simulink model "orbitcom_R20b_finalversion"  (R2020b)
settings: Solver=FixedStepAuto  StartTime=0.0  StopTime=tsimulation  FixedStep=delta_t  RelTol=1e-3
values from neighbouring files (symbols this model uses):
  a = 6678    [linkbudgetuplinkvhf.m]    (also in main_link.m)
  d_0 = (sqrt((R_earth+alt_orbit)^2-R_earth^2))/1000    [linkbudgetuplinkvhf.m]    (also in main_link.m)
  day = 1    [main_link.m]
  delta_t = 0.5    [main_link.m]
  e = 0.001    [main_link.m]
  h = u(1)/1000    [ecef_2_enu.m]    (also in geod_2_ecef.m = u(1); main_link.m = 189)
  hours = 4    [main_link.m]
  i = 51.6    [main_link.m]
  lat = u(2)    [ecef_2_enu.m]    (also in geod_2_ecef.m; main_link.m = 43.6)
  long = u(3)    [ecef_2_enu.m]    (also in geod_2_ecef.m; main_link.m = 1.44)
  m = 10    [main_link.m]
  minutes = 0    [main_link.m]
  month = 1    [main_link.m]
  nu = 0    [main_link.m]
  O = 120    [main_link.m]
  o = 90    [main_link.m]
  seconds = 0    [main_link.m]
  year = 2020    [main_link.m]
undefined symbols (not defined in the file or in its folder): DiscIntNeverNeededParam, km, s
libraries: vrlib x10, aerolibutil x9, aerolibconvert2 x6, sharedtransform x1, My_library x1, simulink_extras x1, aerolibgravity2 x1, aerolibcelestial x1
settings Model: Creator=Ricardo  LastModifiedBy=bouza

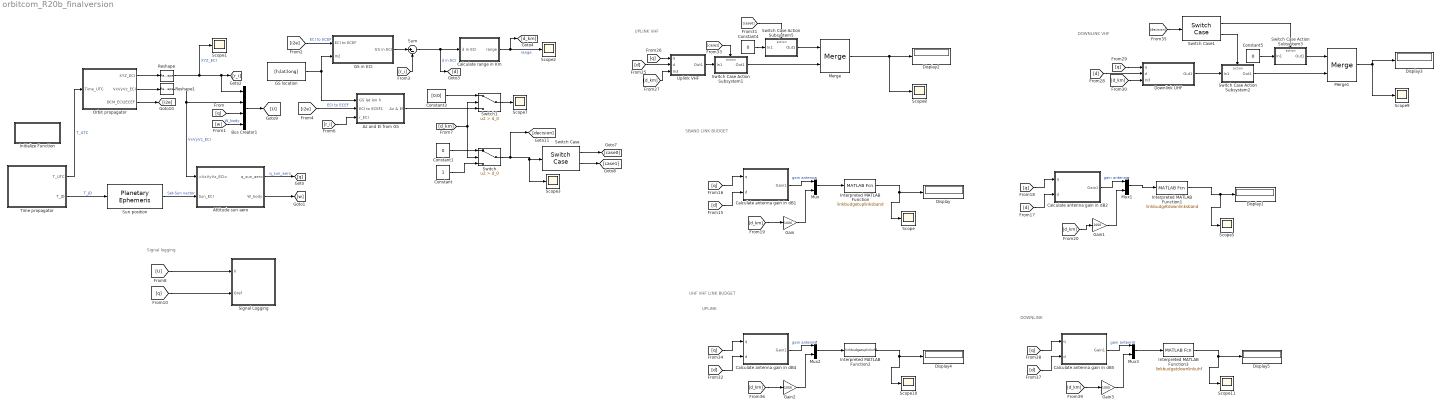
== system orbitcom_R20b_finalversion ==
  note: UHF VHF LINK BUDGET
  note: SBAND LINK BUDGET
  note: UPLINK VHF
  note: Signal logging
  note: DOWNLINK VHF
  note: UPLINK
  note: DOWNLINK
  Attitude sun aero : Subsystem
  Az and El from GS : Subsystem
  Bus Creator1 : BusCreator  Inputs=4
  Calculate antenna gain in dB1 : Subsystem
  Calculate antenna gain in dB2 : Subsystem
  Calculate antenna gain in dB4 : Subsystem
  Calculate antenna gain in dB5 : Subsystem
  Calculate range in Km : Subsystem
  Constant : Constant
  Constant1 : Constant  Value=0
  Constant3 : Constant  Value=[0;0]
  Constant4 : Constant  Value=0
  Constant5 : Constant  Value=0
  Display{,1..5} (6 alike) : Display
  Downlink UHF : Subsystem
  GS in ECI : Subsystem
  GS location : Constant  Value=[h;lat;long]
  Gain{,1..3} (4 alike) : Gain  Gain=1000
  Initialize Function : Subsystem  TreatAsAtomicUnit=on
  Interpreted MATLAB Function : MATLABFcn  MATLABFcn=linkbudgetuplinksband  OutputDimensions=1
  Interpreted MATLAB Function1 : MATLABFcn  MATLABFcn=linkbudgetdownlinksband  OutputDimensions=1
  Interpreted MATLAB Function2 : MATLABFcn  MATLABFcn=linkbudgetuplinkvhf  OutputDimensions=1
  Interpreted MATLAB Function3 : MATLABFcn  MATLABFcn=linkbudgetdownlinkuhf  OutputDimensions=1
  Merge : Merge
  Merge1 : Merge
  Mux{,1..3} (4 alike) : Mux  Inputs=2
  Orbit propagator : Subsystem
  Reshape : Reshape
  Reshape1 : Reshape
  Scope{,1..3,5,7..11} (10 alike) : Scope
  Signal Logging : Subsystem
  Sum : Sum  Inputs=|+-
  Sun position : aerolibcelestial/Planetary Ephemeris  kmflag=km,km/s  epochflag=Julian date  de=DE405  nCenter=Earth  nTarget=Sun  errorflag=Error  velflag=off
      settings: SourceProductBaseCode=AE
  Switch : Switch  Criteria=u2 > Threshold  Threshold=d_0
  Switch Case : SwitchCase  CaseConditions={0, 1}  ShowDefaultCase=off
  Switch Case Action Subsystem1 : Subsystem  TreatAsAtomicUnit=on
  Switch Case Action Subsystem2 : Subsystem  TreatAsAtomicUnit=on
  Switch Case Action Subsystem3 : Subsystem  TreatAsAtomicUnit=on
  Switch Case Action Subsystem5 : Subsystem  TreatAsAtomicUnit=on
  Switch Case1 : SwitchCase  CaseConditions={0, 1}  ShowDefaultCase=off
  Switch1 : Switch  Criteria=u2 > Threshold  Threshold=d_0
  Time propagator : Subsystem
  Uplink VHF : Subsystem
  wires:
  Orbit propagator/2(VxVyVz_ECI) -> Reshape1/1
  Orbit propagator/1(XYZ_ECI) -> Reshape/1
  Sun position/1 -> Attitude sun aero/2(Sun_ECI)  "Sat-Sun vector"
  Time propagator/1(T_UTC) -> Orbit propagator/1("Time_UTC ")  "T_UTC"
  Attitude sun aero/1(q_sun_aero) -> [q]  "q_sun_aero"
  Time propagator/2(T_JD) -> Sun position/1  "T_JD"
  Orbit propagator/3(DCM_ECI2ECEF) -> [i2e]
  Attitude sun aero/2(W_body) -> [w]
  [q] -> Bus Creator1/3
  [w] -> Bus Creator1/4  "W_body"
  Bus Creator1/1 -> [U]
  [q] -> Signal Logging/2(Qref)
  [U] -> Signal Logging/1(U)
  Reshape1/1 -> Bus Creator1/2, Attitude sun aero/1(<VxVyVz_ECI>)  "VxVyVz_ECI"
  Reshape/1 -> Scope1/1, Bus Creator1/1, [r_i]  "XYZ_ECI"
  GS location/1 -> GS in ECI/2(In2), Az and El from GS/1(GS lat lon h)
  Switch/1 -> [decision], Switch Case/1, Scope3/1
  Constant1/1 -> Switch/1
  Constant/1 -> Switch/3
  [r_i] -> Sum/2
  Switch1/1 -> Scope7/1
  [i2e] -> Az and El from GS/2(ECI to ECEF1)  "ECI to ECEF"
  [r_i] -> Az and El from GS/3(r_ECI)
  Constant3/1 -> Switch1/1
  Az and El from GS/1(Az & El) -> Switch1/3
  Calculate range in Km/1(range) -> [d_km], Scope2/1  "range"
  Sum/1 -> Calculate range in Km/1(d in ECI), [d]  "d in ECI"
  [d_km] -> Switch1/2, Switch/2
  [i2e] -> GS in ECI/1(ECI to ECEF)  "ECI to ECEF"
  GS in ECI/1(GS in ECI) -> Sum/1
  [q] -> Calculate antenna gain in dB1/1(q)
  [d] -> Calculate antenna gain in dB1/2(d)
  Interpreted MATLAB Function/1 -> Scope/1, Display/1
  Interpreted MATLAB Function1/1 -> Scope5/1, Display1/1
  [q] -> Calculate antenna gain in dB2/1(q)
  [d] -> Calculate antenna gain in dB2/2(d)
  Calculate antenna gain in dB1/1(Gain1) -> Mux/1  "gain antenna"
  Mux/1 -> Interpreted MATLAB Function/1
  Calculate antenna gain in dB2/1(Gain1) -> Mux1/1  "gain antenna"
  Mux1/1 -> Interpreted MATLAB Function1/1
  [d_km] -> Gain/1
  Gain/1 -> Mux/2
  [d_km] -> Gain1/1
  Gain1/1 -> Mux1/2
  Switch Case/1 -> [case0]
  Constant4/1 -> Switch Case Action Subsystem5/1(In1)
  Switch Case Action Subsystem5/1(Out1) -> Merge/1
  Switch Case Action Subsystem1/1(Out1) -> Merge/2
  [q] -> Uplink VHF/1(q)
  [d] -> Uplink VHF/2(d)
  [d_km] -> Uplink VHF/3(In3)
  Merge/1 -> Scope8/1, Display2/1
  Uplink VHF/1(Out1) -> Switch Case Action Subsystem1/1(In1)
  Switch Case Action Subsystem3/1(Out1) -> Merge1/1
  Merge1/1 -> Scope9/1, Display3/1
  Switch Case Action Subsystem2/1(Out1) -> Merge1/2
  Constant5/1 -> Switch Case Action Subsystem3/1(In1)
  [q] -> Downlink UHF/1(q)
  [d] -> Downlink UHF/2(d)
  [d_km] -> Downlink UHF/3(In3)
  Downlink UHF/1(Out1) -> Switch Case Action Subsystem2/1(In1)
  Switch Case/2 -> [case1]
  [case0] -> Switch Case Action Subsystem5/Action
  Switch Case1/1 -> Switch Case Action Subsystem3/Action
  [case1] -> Switch Case Action Subsystem1/Action
  [decision] -> Switch Case1/1
  Switch Case1/2 -> Switch Case Action Subsystem2/Action
  [d_km] -> Gain2/1
  Mux2/1 -> Interpreted MATLAB Function2/1
  Calculate antenna gain in dB4/1(Gain1) -> Mux2/1  "gain antenna"
  Gain2/1 -> Mux2/2
  Interpreted MATLAB Function2/1 -> Scope10/1, Display4/1
  [q] -> Calculate antenna gain in dB4/1(q)
  [d] -> Calculate antenna gain in dB4/2(d)
  [d_km] -> Gain3/1
  Mux3/1 -> Interpreted MATLAB Function3/1
  Calculate antenna gain in dB5/1(Gain1) -> Mux3/1  "gain antenna"
  Gain3/1 -> Mux3/2
  Interpreted MATLAB Function3/1 -> Scope11/1, Display5/1
  [q] -> Calculate antenna gain in dB5/1(q)
  [d] -> Calculate antenna gain in dB5/2(d)

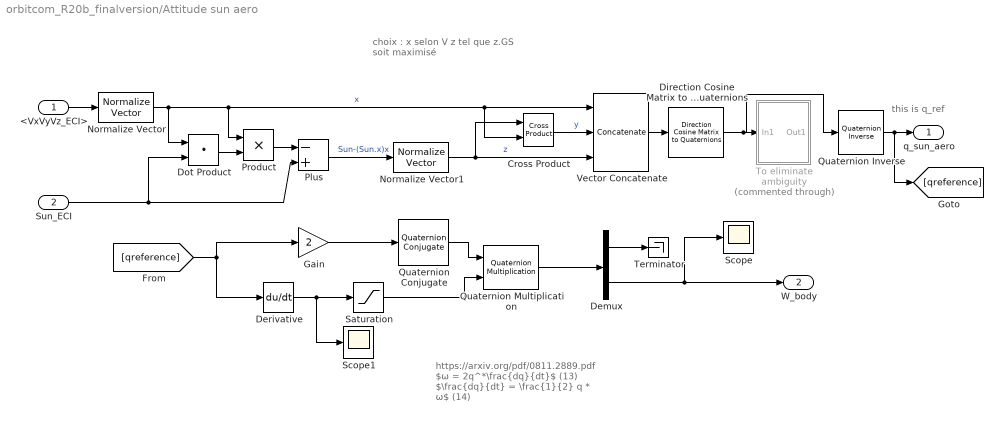
== system orbitcom_R20b_finalversion/Attitude sun aero ==
  note: this is q_ref
  note: choix :
      | x selon V
      | z tel que z.GS soit maximisé
  note: https://arxiv.org/pdf/0811.2889.pdf
      | $ω = 2q^*\frac{dq}{dt}$ (13)
      |
      | $\frac{dq}{dt} = \frac{1}{2} q * ω$ (14)
  <VxVyVz_ECI> : Inport
  Sun_ECI : Inport  Port=2
  Cross Product : vrlib/Utilities/Cross Product
  Demux : Demux  Outputs=[1 3]
  Derivative : Derivative
  Direction Cosine Matrix to Quaternions : sharedtransform/Direction Cosine Matrix  to Quaternions  aMode=0  action=None  tolerance=eps(2)
      settings: SourceProductBaseCode=AE,PW,DR,MT,UV,VE
  Dot Product : DotProduct  InputSameDT=on  OutDataTypeStr=Inherit: Inherit via internal rule
  Gain : Gain  Gain=2
  Normalize Vector : vrlib/Utilities/Normalize Vector  maxzero=0
  Normalize Vector1 : vrlib/Utilities/Normalize Vector  maxzero=0
  Plus : Sum  Inputs=-+
  Product : Product
  Quaternion Conjugate : aerolibutil/Quaternion Conjugate
      settings: SourceProductBaseCode=AE
  Quaternion Inverse : aerolibutil/Quaternion Inverse
  Quaternion Multiplication : aerolibutil/Quaternion Multiplication
  Saturation : Saturate  UpperLimit=5.5e-4  LowerLimit=-5.5e-4
  Scope : Scope
  Scope1 : Scope
  Terminator : Terminator
  To eliminate ambiguity : Subsystem  Commented=through
  Vector Concatenate : Concatenate  NumInputs=3  Mode=Multidimensional array  ConcatenateDimension=2
  q_sun_aero : Outport  VectorParamsAs1DForOutWhenUnconnected=off
  W_body : Outport  Port=2  VectorParamsAs1DForOutWhenUnconnected=off
  wires:
  Quaternion Inverse/1 -> q_sun_aero/1, [qreference]
  Product/1 -> Plus/1
  Dot Product/1 -> Product/2
  Cross Product/1 -> Vector Concatenate/2  "y"
  Normalize Vector1/1 -> Vector Concatenate/3, Cross Product/1  "z"
  Plus/1 -> Normalize Vector1/1  "Sun-(Sun.x)x"
  Sun_ECI/1 -> Dot Product/2, Plus/2
  Vector Concatenate/1 -> Direction Cosine Matrix to Quaternions/1
  Direction Cosine Matrix to Quaternions/1 -> Quaternion Inverse/1, To eliminate ambiguity/1(In1)
  Normalize Vector/1 -> Dot Product/1, Vector Concatenate/1, Cross Product/2, Product/1  "x"
  <VxVyVz_ECI>/1 -> Normalize Vector/1
  [qreference] -> Derivative/1, Gain/1
  Demux/1 -> Terminator/1
  Demux/2 -> W_body/1, Scope/1
  Quaternion Multiplication/1 -> Demux/1
  Quaternion Conjugate/1 -> Quaternion Multiplication/1
  Derivative/1 -> Scope1/1, Saturation/1
  Saturation/1 -> Quaternion Multiplication/2
  Gain/1 -> Quaternion Conjugate/1

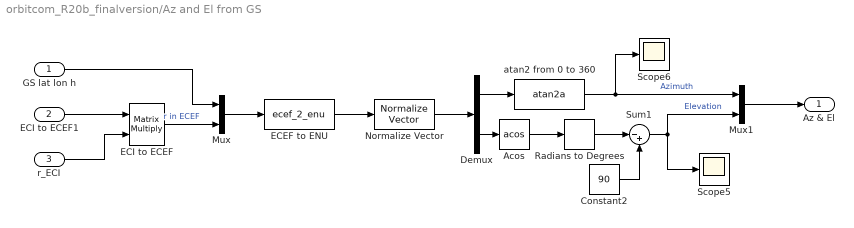
== system orbitcom_R20b_finalversion/Az and El from GS ==
  GS lat lon h : Inport
  ECI to ECEF1 : Inport  Port=2
  r_ECI : Inport  Port=3
  Acos : Trigonometry  Operator=acos
  Constant2 : Constant  Value=90
  Demux : Demux  Outputs=[2,1]
  ECEF to ENU : MATLABFcn  MATLABFcn=ecef_2_enu  OutputDimensions=[3;1]  Output1D=off
  ECI to ECEF : Product  Multiplication=Matrix(*)
  Mux : Mux  Inputs=2
  Mux1 : Mux  Inputs=2
  Normalize Vector : vrlib/Utilities/Normalize Vector  maxzero=0
  Radians to Degrees : simulink_extras/Transformations/Radians to Degrees
  Scope5 : Scope
  Scope6 : Scope
  Sum1 : Sum  Inputs=|-+
  atan2 from 0 to 360 : MATLABFcn  MATLABFcn=atan2a
  Az & El : Outport
  wires:
  atan2 from 0 to 360/1 -> Scope6/1, Mux1/1  "Azimuth"
  ECEF to ENU/1 -> Normalize Vector/1
  GS lat lon h/1 -> Mux/1
  Acos/1 -> Radians to Degrees/1
  ECI to ECEF1/1 -> ECI to ECEF/1
  ECI to ECEF/1 -> Mux/2  "r in ECEF"
  Demux/2 -> Acos/1
  Mux/1 -> ECEF to ENU/1
  Sum1/1 -> Scope5/1, Mux1/2  "Elevation"
  Normalize Vector/1 -> Demux/1
  Demux/1 -> atan2 from 0 to 360/1
  Radians to Degrees/1 -> Sum1/1
  Constant2/1 -> Sum1/2
  r_ECI/1 -> ECI to ECEF/2
  Mux1/1 -> Az & El/1

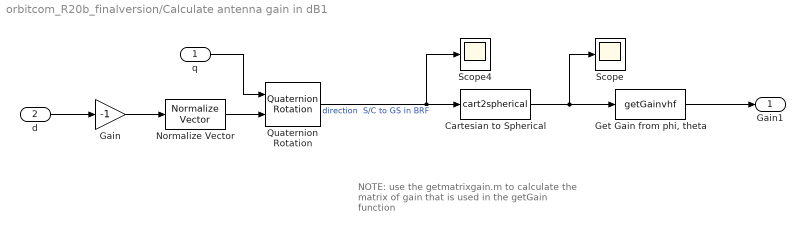
== system orbitcom_R20b_finalversion/Calculate antenna gain in dB1 ==
  note: NOTE: use the getmatrixgain.m to calculate
      | the matrix of gain that is used in the getGain
      | function
  q : Inport
  d : Inport  Port=2
  Cartesian to Spherical : MATLABFcn  MATLABFcn=cart2spherical
  Gain : Gain  Gain=-1
  "Get Gain from phi, theta" : MATLABFcn  MATLABFcn=getGainvhf
  Normalize Vector : vrlib/Utilities/Normalize Vector  maxzero=0
  Quaternion Rotation : aerolibutil/Quaternion Rotation
  Scope : Scope
  Scope4 : Scope
  Gain1 : Outport
  wires:
  d/1 -> Gain/1
  Gain/1 -> Normalize Vector/1
  Cartesian to Spherical/1 -> "Get Gain from phi, theta"/1, Scope/1
  q/1 -> Quaternion Rotation/1
  Normalize Vector/1 -> Quaternion Rotation/2
  Quaternion Rotation/1 -> Cartesian to Spherical/1, Scope4/1  "direction  S/C to GS in BRF"
  "Get Gain from phi, theta"/1 -> Gain1/1

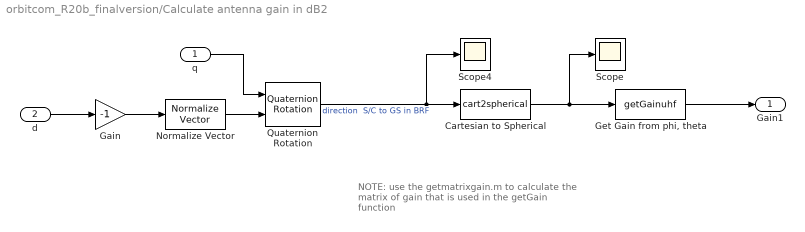
== system orbitcom_R20b_finalversion/Calculate antenna gain in dB2 ==
  note: NOTE: use the getmatrixgain.m to calculate
      | the matrix of gain that is used in the getGain
      | function
  q : Inport
  d : Inport  Port=2
  Cartesian to Spherical : MATLABFcn  MATLABFcn=cart2spherical
  Gain : Gain  Gain=-1
  "Get Gain from phi, theta" : MATLABFcn  MATLABFcn=getGainuhf
  Normalize Vector : vrlib/Utilities/Normalize Vector  maxzero=0
  Quaternion Rotation : aerolibutil/Quaternion Rotation
  Scope : Scope
  Scope4 : Scope
  Gain1 : Outport
  wires:
  d/1 -> Gain/1
  Gain/1 -> Normalize Vector/1
  Cartesian to Spherical/1 -> "Get Gain from phi, theta"/1, Scope/1
  q/1 -> Quaternion Rotation/1
  Normalize Vector/1 -> Quaternion Rotation/2
  Quaternion Rotation/1 -> Cartesian to Spherical/1, Scope4/1  "direction  S/C to GS in BRF"
  "Get Gain from phi, theta"/1 -> Gain1/1

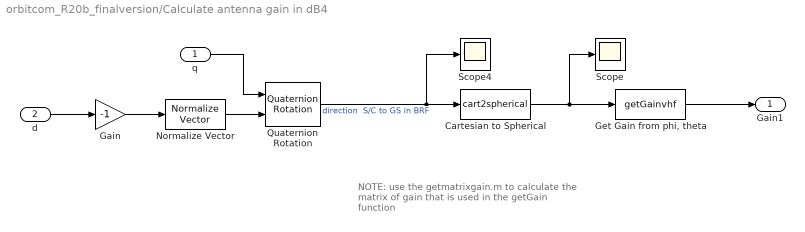
== system orbitcom_R20b_finalversion/Calculate antenna gain in dB4 ==
  note: NOTE: use the getmatrixgain.m to calculate
      | the matrix of gain that is used in the getGain
      | function
  q : Inport
  d : Inport  Port=2
  Cartesian to Spherical : MATLABFcn  MATLABFcn=cart2spherical
  Gain : Gain  Gain=-1
  "Get Gain from phi, theta" : MATLABFcn  MATLABFcn=getGainvhf
  Normalize Vector : vrlib/Utilities/Normalize Vector  maxzero=0
  Quaternion Rotation : aerolibutil/Quaternion Rotation
  Scope : Scope
  Scope4 : Scope
  Gain1 : Outport
  wires:
  d/1 -> Gain/1
  Gain/1 -> Normalize Vector/1
  Cartesian to Spherical/1 -> "Get Gain from phi, theta"/1, Scope/1
  q/1 -> Quaternion Rotation/1
  Normalize Vector/1 -> Quaternion Rotation/2
  Quaternion Rotation/1 -> Cartesian to Spherical/1, Scope4/1  "direction  S/C to GS in BRF"
  "Get Gain from phi, theta"/1 -> Gain1/1

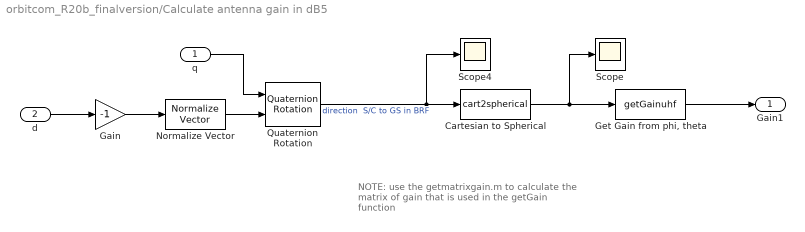
== system orbitcom_R20b_finalversion/Calculate antenna gain in dB5 ==
  note: NOTE: use the getmatrixgain.m to calculate
      | the matrix of gain that is used in the getGain
      | function
  q : Inport
  d : Inport  Port=2
  Cartesian to Spherical : MATLABFcn  MATLABFcn=cart2spherical
  Gain : Gain  Gain=-1
  "Get Gain from phi, theta" : MATLABFcn  MATLABFcn=getGainuhf
  Normalize Vector : vrlib/Utilities/Normalize Vector  maxzero=0
  Quaternion Rotation : aerolibutil/Quaternion Rotation
  Scope : Scope
  Scope4 : Scope
  Gain1 : Outport
  wires:
  d/1 -> Gain/1
  Gain/1 -> Normalize Vector/1
  Cartesian to Spherical/1 -> "Get Gain from phi, theta"/1, Scope/1
  q/1 -> Quaternion Rotation/1
  Normalize Vector/1 -> Quaternion Rotation/2
  Quaternion Rotation/1 -> Cartesian to Spherical/1, Scope4/1  "direction  S/C to GS in BRF"
  "Get Gain from phi, theta"/1 -> Gain1/1

== system orbitcom_R20b_finalversion/Calculate range in Km ==
  d in ECI : Inport
  Dot Product : DotProduct  InputSameDT=on  OutDataTypeStr=Inherit: Inherit via internal rule
  Gain : Gain  Gain=1/1000
  Sqrt : Sqrt  SaturateOnIntegerOverflow=on
  range : Outport
  wires:
  Gain/1 -> range/1
  Sqrt/1 -> Gain/1
  Dot Product/1 -> Sqrt/1
  d in ECI/1 -> Dot Product/1, Dot Product/2

== system orbitcom_R20b_finalversion/Downlink UHF ==
  q : Inport
  d : Inport  Port=2
  In3 : Inport  Port=3
  Calculate antenna gain in dB4 : Subsystem
  Gain2 : Gain  Gain=1000
  Interpreted MATLAB Function2 : MATLABFcn  MATLABFcn=linkbudgetdownlinkuhf  OutputDimensions=1
  Mux2 : Mux  Inputs=2
  Out1 : Outport
  wires:
  Mux2/1 -> Interpreted MATLAB Function2/1
  Gain2/1 -> Mux2/2
  q/1 -> Calculate antenna gain in dB4/1(q)
  Calculate antenna gain in dB4/1(Gain1) -> Mux2/1  "gain antenna"
  Interpreted MATLAB Function2/1 -> Out1/1
  d/1 -> Calculate antenna gain in dB4/2(d)
  In3/1 -> Gain2/1

== system orbitcom_R20b_finalversion/GS in ECI ==
  ECI to ECEF : Inport
  In2 : Inport  Port=2
  ECEF to ECI : Product  Multiplication=Matrix(*)
  Geod to ECEF : MATLABFcn  MATLABFcn=geod_2_ecef  OutputDimensions=[3;1]  Output1D=off
  Permute Dimensions : PermuteDimensions
  Scope : Scope
  GS in ECI : Outport
  wires:
  ECI to ECEF/1 -> Permute Dimensions/1
  Permute Dimensions/1 -> ECEF to ECI/1
  ECEF to ECI/1 -> GS in ECI/1, Scope/1  "GS in ECI"
  In2/1 -> Geod to ECEF/1
  Geod to ECEF/1 -> ECEF to ECI/2

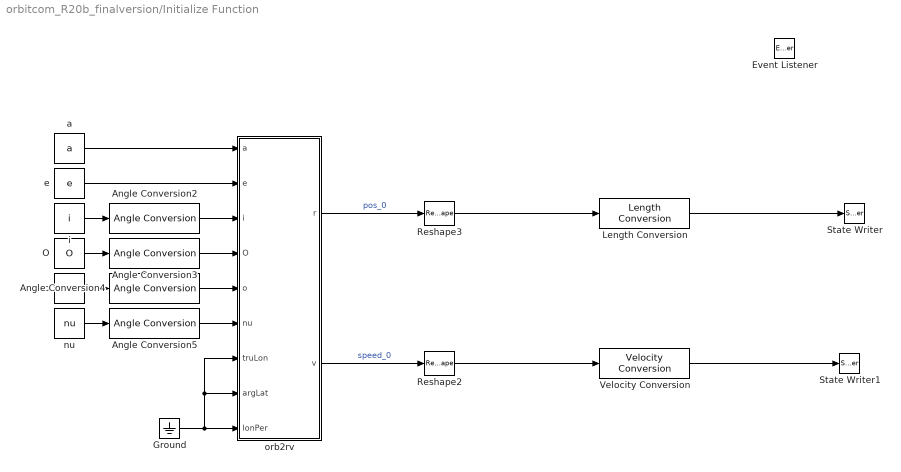
== system orbitcom_R20b_finalversion/Initialize Function ==
  Angle Conversion{2..5} (4 alike) : aerolibconvert2/Angle Conversion  IU=deg  OU=rad
  Event Listener : EventListener  DisableCoverage=on  EventName=reset
  Ground : Ground
  Length Conversion : aerolibconvert2/Length Conversion  IU=km  OU=m
  O : Constant  Value=O
  Reshape2 : Reshape  OutputDimensionality=Column vector (2-D)
  Reshape3 : Reshape  OutputDimensionality=Column vector (2-D)
  State Writer : StateWriter  StateOwnerBlock=../../Orbit propagator/Integrator_pos
  State Writer1 : StateWriter  StateOwnerBlock=../../Orbit propagator/Integrator_speed
  Velocity Conversion : aerolibconvert2/Velocity Conversion  IU=km/s  OU=m/s
  a : Constant  Value=a
  e : Constant  Value=e
  i : Constant  Value=i
  nu : Constant  Value=nu
  o : Constant  Value=o
  orb2rv : MATLAB Function  TreatAsAtomicUnit=on
  wires:
  Angle Conversion2/1 -> orb2rv/3(i)
  Length Conversion/1 -> State Writer/1
  Angle Conversion4/1 -> orb2rv/5(o)
  nu/1 -> Angle Conversion5/1
  Angle Conversion3/1 -> orb2rv/4(O)
  e/1 -> orb2rv/2(e)
  Reshape3/1 -> Length Conversion/1
  O/1 -> Angle Conversion3/1
  a/1 -> orb2rv/1(a)
  i/1 -> Angle Conversion2/1
  orb2rv/1(r) -> Reshape3/1  "pos_0"
  o/1 -> Angle Conversion4/1
  Angle Conversion5/1 -> orb2rv/6(nu)
  Velocity Conversion/1 -> State Writer1/1
  Reshape2/1 -> Velocity Conversion/1
  orb2rv/2(v) -> Reshape2/1  "speed_0"
  Ground/1 -> orb2rv/8(argLat), orb2rv/7(truLon), orb2rv/9(lonPer)

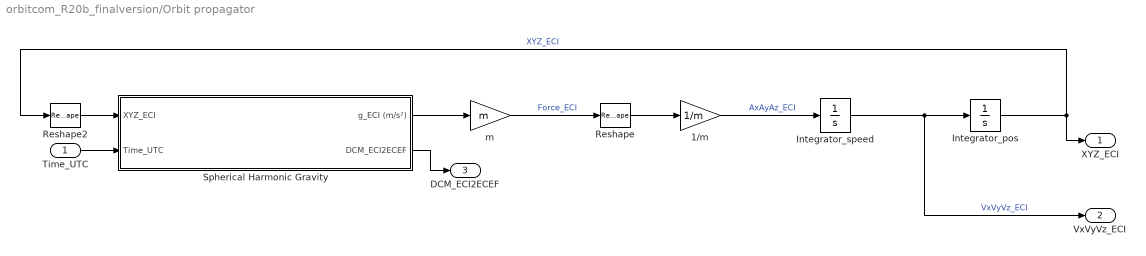
== system orbitcom_R20b_finalversion/Orbit propagator ==
  "Time_UTC " : Inport
  1/m : Gain  Gain=1/m
  Integrator_pos : Integrator
  Integrator_speed : Integrator
  Reshape : Reshape  OutputDimensionality=Column vector (2-D)
  Reshape2 : Reshape  OutputDimensionality=Column vector (2-D)
  Spherical Harmonic Gravity : Subsystem  TreatAsAtomicUnit=on  SystemSampleTime=1
  m : Gain  Gain=m
  XYZ_ECI : Outport  VectorParamsAs1DForOutWhenUnconnected=off
  VxVyVz_ECI : Outport  Port=2
  DCM_ECI2ECEF : Outport  Port=3
  wires:
  Integrator_pos/1 -> Reshape2/1, XYZ_ECI/1  "XYZ_ECI"
  Integrator_speed/1 -> VxVyVz_ECI/1, Integrator_pos/1  "VxVyVz_ECI"
  1/m/1 -> Integrator_speed/1  "AxAyAz_ECI"
  Reshape/1 -> 1/m/1
  m/1 -> Reshape/1  "Force_ECI"
  Spherical Harmonic Gravity/1(g_ECI (m/s²)) -> m/1
  "Time_UTC "/1 -> Spherical Harmonic Gravity/2(Time_UTC)
  Reshape2/1 -> Spherical Harmonic Gravity/1(XYZ_ECI)
  Spherical Harmonic Gravity/2(DCM_ECI2ECEF) -> DCM_ECI2ECEF/1

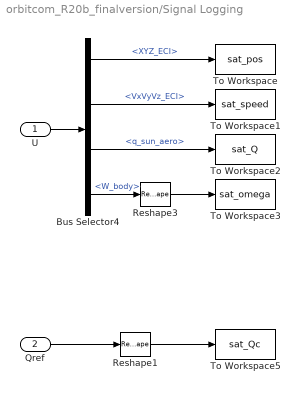
== system orbitcom_R20b_finalversion/Signal Logging ==
  U : Inport
  Qref : Inport  Port=2
  Bus Selector4 : BusSelector  OutputSignals=XYZ_ECI,VxVyVz_ECI,q_sun_aero,W_body
  Reshape1 : Reshape
  Reshape3 : Reshape
  To Workspace : ToWorkspace  VariableName=sat_pos  SaveFormat=Timeseries  SampleTime=1
      settings: Save2DSignal=2-D array (concatenate along first dimension)
  To Workspace1 : ToWorkspace  VariableName=sat_speed  SaveFormat=Timeseries  SampleTime=1
      settings: Save2DSignal=2-D array (concatenate along first dimension)
  To Workspace2 : ToWorkspace  VariableName=sat_Q  SaveFormat=Timeseries  SampleTime=1
      settings: Save2DSignal=2-D array (concatenate along first dimension)
  To Workspace3 : ToWorkspace  VariableName=sat_omega  SaveFormat=Timeseries  SampleTime=1
      settings: Save2DSignal=2-D array (concatenate along first dimension)
  To Workspace5 : ToWorkspace  VariableName=sat_Qc  SaveFormat=Timeseries  SampleTime=1
      settings: Save2DSignal=2-D array (concatenate along first dimension)
  wires:
  Bus Selector4/3 -> To Workspace2/1  "<q_sun_aero>"
  Bus Selector4/4 -> Reshape3/1  "<W_body>"
  U/1 -> Bus Selector4/1
  Bus Selector4/2 -> To Workspace1/1  "<VxVyVz_ECI>"
  Bus Selector4/1 -> To Workspace/1  "<XYZ_ECI>"
  Qref/1 -> Reshape1/1
  Reshape1/1 -> To Workspace5/1
  Reshape3/1 -> To Workspace3/1

== system orbitcom_R20b_finalversion/Switch Case Action Subsystem1 ==
  In1 : Inport
  Action Port : ActionPort  ActionPortLabel=case [ 1 ]:
  Out1 : Outport  VectorParamsAs1DForOutWhenUnconnected=off
  wires:
  In1/1 -> Out1/1

== system orbitcom_R20b_finalversion/Switch Case Action Subsystem2 ==
  In1 : Inport
  Action Port : ActionPort  ActionPortLabel=case [ 1 ]:
  Out1 : Outport  VectorParamsAs1DForOutWhenUnconnected=off
  wires:
  In1/1 -> Out1/1

== system orbitcom_R20b_finalversion/Switch Case Action Subsystem3 ==
  In1 : Inport
  Action Port : ActionPort  ActionPortLabel=case [ 0 ]:
  Out1 : Outport  VectorParamsAs1DForOutWhenUnconnected=off
  wires:
  In1/1 -> Out1/1

== system orbitcom_R20b_finalversion/Switch Case Action Subsystem5 ==
  In1 : Inport
  Action Port : ActionPort  ActionPortLabel=case [ 0 ]:
  Out1 : Outport  VectorParamsAs1DForOutWhenUnconnected=off
  wires:
  In1/1 -> Out1/1

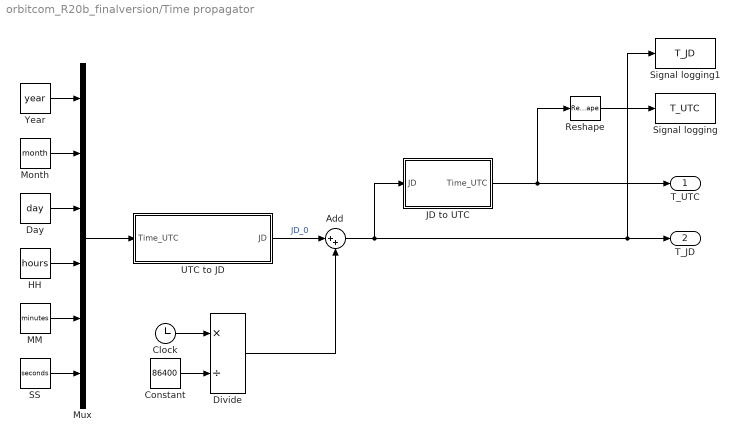
== system orbitcom_R20b_finalversion/Time propagator ==
  Add : Sum  Inputs=|++
  Clock : Clock
  Constant : Constant  Value=86400
  Day : Constant  Value=day
  Divide : Product  Inputs=*/
  HH : Constant  Value=hours
  JD to UTC : MATLAB Function  TreatAsAtomicUnit=on
  MM : Constant  Value=minutes
  Month : Constant  Value=month
  Mux : Mux  Inputs=6
  Reshape : Reshape
  SS : Constant  Value=seconds
  Signal logging : ToWorkspace  VariableName=T_UTC  SaveFormat=Timeseries  SampleTime=1
      settings: Save2DSignal=2-D array (concatenate along first dimension)
  Signal logging1 : ToWorkspace  VariableName=T_JD  SaveFormat=Timeseries  SampleTime=1
      settings: Save2DSignal=2-D array (concatenate along first dimension)
  UTC to JD : MATLAB Function  TreatAsAtomicUnit=on
  Year : Constant  Value=year
  T_UTC : Outport  VectorParamsAs1DForOutWhenUnconnected=off
  T_JD : Outport  Port=2  VectorParamsAs1DForOutWhenUnconnected=off
  wires:
  UTC to JD/1(JD) -> Add/1  "JD_0"
  Clock/1 -> Divide/1
  Constant/1 -> Divide/2
  JD to UTC/1(Time_UTC) -> T_UTC/1, Reshape/1
  Divide/1 -> Add/2
  Mux/1 -> UTC to JD/1(Time_UTC)
  Day/1 -> Mux/3
  Month/1 -> Mux/2
  Year/1 -> Mux/1
  HH/1 -> Mux/4
  MM/1 -> Mux/5
  SS/1 -> Mux/6
  Reshape/1 -> Signal logging/1
  Add/1 -> Signal logging1/1, T_JD/1, JD to UTC/1(JD)

== system orbitcom_R20b_finalversion/Uplink VHF ==
  q : Inport
  d : Inport  Port=2
  In3 : Inport  Port=3
  Calculate antenna gain in dB4 : Subsystem
  Gain2 : Gain  Gain=1000
  Interpreted MATLAB Function2 : MATLABFcn  MATLABFcn=linkbudgetuplinkvhf  OutputDimensions=1
  Mux2 : Mux  Inputs=2
  Scope : Scope
  Out1 : Outport
  wires:
  Gain2/1 -> Mux2/2
  In3/1 -> Gain2/1
  Interpreted MATLAB Function2/1 -> Out1/1
  Mux2/1 -> Interpreted MATLAB Function2/1
  Calculate antenna gain in dB4/1(Gain1) -> Scope/1, Mux2/1  "gain antenna"
  d/1 -> Calculate antenna gain in dB4/2(d)
  q/1 -> Calculate antenna gain in dB4/1(q)

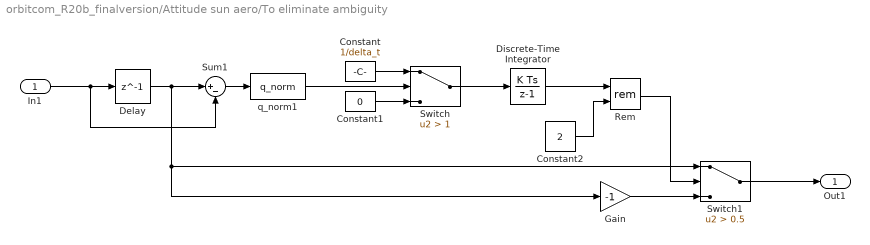
== system orbitcom_R20b_finalversion/Attitude sun aero/To eliminate ambiguity ==
  In1 : Inport
  Constant : Constant  Value=1/delta_t
  Constant1 : Constant  Value=0
  Constant2 : Constant  Value=2
  Delay : Delay  DelayLength=1
  Discrete-Time Integrator : DiscreteIntegrator  SampleTime=-1  ICPrevOutput=DiscIntNeverNeededParam  ICPrevScaledInput=DiscIntNeverNeededParam
  Gain : Gain  Gain=-1
  Rem : Math  Operator=rem  SaturateOnIntegerOverflow=on
  Sum1 : Sum  Inputs=|+-
  Switch : Switch  Criteria=u2 > Threshold  Threshold=1
  Switch1 : Switch  Criteria=u2 > Threshold  Threshold=0.5
  q_norm1 : My_library/q_norm
      settings: SourceProductName=My Library
  Out1 : Outport
  wires:
  Delay/1 -> Gain/1, Switch1/1, Sum1/1
  Sum1/1 -> q_norm1/1
  q_norm1/1 -> Switch/2
  Switch/1 -> Discrete-Time Integrator/1
  Constant/1 -> Switch/1
  Constant1/1 -> Switch/3
  In1/1 -> Sum1/2, Delay/1
  Discrete-Time Integrator/1 -> Rem/1
  Constant2/1 -> Rem/2
  Rem/1 -> Switch1/2
  Gain/1 -> Switch1/3
  Switch1/1 -> Out1/1

== system orbitcom_R20b_finalversion/Downlink UHF/Calculate antenna gain in dB4 ==
  note: NOTE: use the getmatrixgain.m to calculate
      | the matrix of gain that is used in the getGain
      | function
  q : Inport
  d : Inport  Port=2
  Cartesian to Spherical : MATLABFcn  MATLABFcn=cart2spherical
  Gain : Gain  Gain=-1
  "Get Gain from phi, theta" : MATLABFcn  MATLABFcn=getGainuhf
  Normalize Vector : vrlib/Utilities/Normalize Vector  maxzero=0
  Quaternion Rotation : aerolibutil/Quaternion Rotation
  Scope : Scope
  Scope4 : Scope
  Gain1 : Outport
  wires:
  d/1 -> Gain/1
  Gain/1 -> Normalize Vector/1
  Cartesian to Spherical/1 -> "Get Gain from phi, theta"/1, Scope/1
  q/1 -> Quaternion Rotation/1
  Normalize Vector/1 -> Quaternion Rotation/2
  Quaternion Rotation/1 -> Cartesian to Spherical/1, Scope4/1  "direction  S/C to GS in BRF"
  "Get Gain from phi, theta"/1 -> Gain1/1

== system orbitcom_R20b_finalversion/Orbit propagator/Spherical Harmonic Gravity ==
  note: Slower subsytem because it's too slow
  XYZ_ECI : Inport
  Time_UTC : Inport  Port=2
  ECI_2_ECEF : MATLABFcn  MATLABFcn=eci2ecef  OutputDimensions=[3,3]  Output1D=off
  Product : Product  Multiplication=Matrix(*)
  Product1 : Product  Inputs=/*  Multiplication=Matrix(*)
  Spherical Harmonic Gravity Model : aerolibgravity2/Spherical Harmonic Gravity Model  units=Metric (MKS)  degree=100  action=Warning  ptype=EGM2008  datafile=''''aerogmm2b.mat''''
      settings: SourceProductBaseCode=AE
  Transpose : Math  Operator=transpose  SignedPower=on  SaturateOnIntegerOverflow=on
  g_ECI (m/s²) : Outport
  DCM_ECI2ECEF : Outport  Port=2
  wires:
  ECI_2_ECEF/1 -> DCM_ECI2ECEF/1, Product1/1, Product/1
  Transpose/1 -> Product1/2
  Product/1 -> Spherical Harmonic Gravity Model/1
  Spherical Harmonic Gravity Model/1 -> Transpose/1
  XYZ_ECI/1 -> Product/2
  Product1/1 -> g_ECI (m/s²)/1
  Time_UTC/1 -> ECI_2_ECEF/1

== system orbitcom_R20b_finalversion/Uplink VHF/Calculate antenna gain in dB4 ==
  note: NOTE: use the getmatrixgain.m to calculate
      | the matrix of gain that is used in the getGain
      | function
  q : Inport
  d : Inport  Port=2
  Cartesian to Spherical : MATLABFcn  MATLABFcn=cart2spherical
  Gain : Gain  Gain=-1
  "Get Gain from phi, theta" : MATLABFcn  MATLABFcn=getGainvhf
  Normalize Vector : vrlib/Utilities/Normalize Vector  maxzero=0
  Quaternion Rotation : aerolibutil/Quaternion Rotation
  Scope : Scope
  Scope4 : Scope
  Gain1 : Outport
  wires:
  d/1 -> Gain/1
  Gain/1 -> Normalize Vector/1
  Cartesian to Spherical/1 -> "Get Gain from phi, theta"/1, Scope/1
  q/1 -> Quaternion Rotation/1
  Normalize Vector/1 -> Quaternion Rotation/2
  Quaternion Rotation/1 -> Cartesian to Spherical/1, Scope4/1  "direction  S/C to GS in BRF"
  "Get Gain from phi, theta"/1 -> Gain1/1

== matlab function orbitcom_R20b_finalversion/Time propagator/JD to UTC ==
  data: JD input; Time_UTC output
function Time_UTC = fcn(JD)
    coder.extrinsic('datetime','datevec');
    Time_UTC = [0,0,0,0,0,0];
Time_UTC =  datevec(datetime(JD,'convertfrom','juliandate'));

== matlab function orbitcom_R20b_finalversion/Time propagator/UTC to JD ==
  data: Time_UTC input; JD output
function JD = fcn(Time_UTC)

% JD = juliandate(Time_UTC);
JD = Dt2jD(Time_UTC);

== matlab function orbitcom_R20b_finalversion/Initialize Function/orb2rv ==
  data: a input; r output; e input; i input; O input; o input; nu input; v output; truLon input; argLat input; lonPer input
%----------------------- Begin Code Sequence -----------------------------%
% Purpose:                                                                %
% Convert a given set of Keplerian Orbital Elements to state vectors in   %
% in the ECI frame of reference                                           %
%                                                                         %
%-------------------------------------------------------------------------%
%                                                                         %
% Inputs:                                                                 %
%-------- 
%a                      [1 x N]                         Semimajor axis
%                                                       (km)
%
%e                      [1 x N]                         Eccentricity Magnitude
%                                                       (unitless)
%
%i                      [1 x N]                         inclination
%                                                       (radians)
%
%O                      [1 x N]                         Right Ascention of
%                                                       the ascending node
%                                                       (radians)
%
%o                      [1 x N]                         Argument of perigee
%                                                       (radians)
%
%nu                     [1 x N]                         True Anomaly
%                                                       (radians)
%
%truLon                 [1 x N]                         True Longitude
%                                                       (radians)
%
%argLat                 [1 x N]                         Argument of Latitude
%                                                       (radians)
%
%lonPer                 [1 x N]                         Longitude of Periapse
%                                                       (radians)
%
%mu                     double                          Gravitational Constant
%                                                       Defaults to Earth if
%                                                       not specified
%
% Outputs:
%---------                                                                %
%r_ECI                  [3 x N]                         Position Vector in
%                                                       ECI coordinate
%                                                       frame of reference
%
%v_ECI                  [3 x N]                         Velocity vector in
%                                                       ECI coordinate
%                                                       frame of reference
%
% References:
%-------------
%Vallado,D. Fundamentals of Astrodynamics and Applications. 2007.
%
% Function Dependencies:
%------------------
%None
%------------------------------------------------------------------       %
% Programed by Darin Koblick  03-04-2012                                  %
%------------------------------------------------------------------       %
function [r,v] = orb2rv(a,e,i,O,o,nu,truLon,argLat,lonPer)
mu = 398600.4418;
%Make all inputs consistent w/ dimensions
a = a(:); e = e(:); i = i(:); O = O(:); o = o(:); nu = nu(:);
if e<1
    p=a*(1-e*e);
else
    p=2*a;
end
ietol = 1e-8;
idx = e < ietol & mod(i,pi) < ietol;
if any(idx); o(idx) = 0; O(idx) = 0; nu(idx) = truLon(idx); end
idx = e < ietol & mod(i,pi) > ietol;
if any(idx); o(idx) = 0; nu(idx) = argLat(idx); end
idx = e > ietol & mod(i,pi) < ietol;
if any(idx); O(idx) = 0; o(idx) = lonPer(idx); end
%Find rPQW and vPQW
rPQW = cat(2,p.*cos(nu)./(1 +e.*cos(nu)),p.*sin(nu)./(1+e.*cos(nu)),zeros(size(nu)));
vPQW = cat(2,-sqrt(mu./p).*sin(nu),sqrt(mu./p).*(e+cos(nu)),zeros(size(nu)));
%Create Transformation Matrix
PQW2IJK = NaN(3,3,size(p,1));
cO = cos(O); sO = sin(O); co = cos(o); so = sin(o); ci = cos(i); si = sin(i);
PQW2IJK(1,1,:) = cO.*co-sO.*so.*ci; PQW2IJK(1,2,:) = -cO.*so-sO.*co.*ci; PQW2IJK(1,3,:) = sO.*si;
PQW2IJK(2,1,:) = sO.*co+cO.*so.*ci; PQW2IJK(2,2,:) = -sO.*so+cO.*co.*ci; PQW2IJK(2,3,:) = -cO.*si;
PQW2IJK(3,1,:) = so.*si;            PQW2IJK(3,2,:) = co.*si;             PQW2IJK(3,3,:) = ci;
%Transform rPQW and vPQW to rECI and vECI
r = multiDimMatrixMultiply(PQW2IJK,rPQW)';  
v = multiDimMatrixMultiply(PQW2IJK,vPQW)';
end
function c = multiDimMatrixMultiply(a,b)
c = NaN(size(b));
c(:,1) = sum(bsxfun(@times,a(1,:,:),permute(b,[3 2 1])),2);
c(:,2) = sum(bsxfun(@times,a(2,:,:),permute(b,[3 2 1])),2);
c(:,3) = sum(bsxfun(@times,a(3,:,:),permute(b,[3 2 1])),2);
end
